simulink model "point_cloud_fusion_node_debag"  (R2021b)
settings: Solver=FixedStepAuto  StartTime=0.0  StopTime=10.0  RelTol=1e-3
model workspace (MAT data in the model file):
  Logfile_Data_Object = ros2bag
  Logfile_Data_Object.FilePath = 'C:\azumiken\lidars_point_raw\lidars_point_raw_0.db3'
  Logfile_Data_Object.StartTime = 1633675920681641206
  Logfile_Data_Object.EndTime = 1633676017682751873
  Logfile_Data_Object.AvailableTopics = table
  Logfile_Data_Object.AvailableTopics.data{1} = [969; 970]
  Logfile_Data_Object.AvailableTopics.data{2} = categorical
  Logfile_Data_Object.AvailableTopics.data{2}.categoryNames = {'sensor_msgs/PointCloud2'}
  Logfile_Data_Object.AvailableTopics.data{2}.codes = [1; 1]
  Logfile_Data_Object.AvailableTopics.data{3}{1} = '% contain additional information such as normals, intensity, etc. The
    | % point data is stored as a binary blob, its layout described by the
    | % contents of the "fields" array.
    | %
    | % The point cloud data may be organized 2d (image-like) or 1d (unordered).
    | % Point clouds organized as 2d images may be produced by camera depth sensors
    | % such as stereo or Time-of-flight.
    | 
    | % Time of sensor data acquisition, and the coordinate frame ID (for 3d points).
    | std_msgs/Header header
    | 
    | % 2D structure of the point cloud. If the cloud is unordered, height is
    | % 1 and width is the length of the point cloud.
    | uint32 height
    | uint32 width
    | 
    | % Describes the channels and their layout in the binary data blob.
    | PointField[] fields
    | 
    | logical    is_bigendian % Is this data bigendian?
    | uint32  point_step      % Length of a point in bytes
    | uint32  row_step        % Length of a row in bytes
    | uint8[] data            % Actual point data, size is (row_step*height)
    | 
    | logical is_dense        % True if there are no invalid points'
  Logfile_Data_Object.AvailableTopics.data{3}{2} = '% contain additional information such as normals, intensity, etc. The
    | % point data is stored as a binary blob, its layout described by the
    | % contents of the "fields" array.
    | %
    | % The point cloud data may be organized 2d (image-like) or 1d (unordered).
    | % Point clouds organized as 2d images may be produced by camera depth sensors
    | % such as stereo or Time-of-flight.
    | 
    | % Time of sensor data acquisition, and the coordinate frame ID (for 3d points).
    | std_msgs/Header header
    | 
    | % 2D structure of the point cloud. If the cloud is unordered, height is
    | % 1 and width is the length of the point cloud.
    | uint32 height
    | uint32 width
    | 
    | % Describes the channels and their layout in the binary data blob.
    | PointField[] fields
    | 
    | logical    is_bigendian % Is this data bigendian?
    | uint32  point_step      % Length of a point in bytes
    | uint32  row_step        % Length of a row in bytes
    | uint8[] data            % Actual point data, size is (row_step*height)
    | 
    | logical is_dense        % True if there are no invalid points'
  Logfile_Data_Object.AvailableTopics.ndims = 2
  Logfile_Data_Object.AvailableTopics.nrows = 2
  Logfile_Data_Object.AvailableTopics.rownames = {'/lidar_front/points_raw'; '/lidar_rear/points_raw'}
  Logfile_Data_Object.AvailableTopics.nvars = 3
  Logfile_Data_Object.AvailableTopics.varnames = {'NumMessages', 'MessageType', 'MessageDefinition'}
  Logfile_Data_Object.AvailableTopics.props.useVariableNamesOriginal = 0
  Logfile_Data_Object.AvailableTopics.props.useDimensionNamesOriginal = 0
  Logfile_Data_Object.AvailableTopics.props.CustomProps = struct()
  Logfile_Data_Object.AvailableTopics.props.VariableCustomProps = struct()
  Logfile_Data_Object.AvailableTopics.props.versionSavedFrom = 4
  Logfile_Data_Object.AvailableTopics.props.minCompatibleVersion = 1
  Logfile_Data_Object.AvailableTopics.props.incompatibilityMsg = ''
  Logfile_Data_Object.AvailableTopics.props.VersionSavedFrom = 4
  Logfile_Data_Object.AvailableTopics.props.Description = ''
  Logfile_Data_Object.AvailableTopics.props.VariableNamesOriginal = {}
  Logfile_Data_Object.AvailableTopics.props.DimensionNames = {'Row', 'Variables'}
  Logfile_Data_Object.AvailableTopics.props.DimensionNamesOriginal = {}
  Logfile_Data_Object.AvailableTopics.props.UserData = []
  Logfile_Data_Object.AvailableTopics.props.VariableDescriptions = {}
  Logfile_Data_Object.AvailableTopics.props.VariableUnits = {}
  Logfile_Data_Object.AvailableTopics.props.VariableContinuity = {}
  Logfile_Data_Object.MessageList = table
  Logfile_Data_Object.MessageList.data{1} = [1633675920681641206 1633675920704850047 1633675920710280571 1633675920841302537 1633675920849007917 1633675920944718285 1633675920950454411 1633675921046456357 1633675921051238695 1633675921143527086 1633675921154682295 1633675921262758351 ... (1939 elements, 1939x1)]
  Logfile_Data_Object.MessageList.data{2} = categorical
  Logfile_Data_Object.MessageList.data{2}.categoryNames = {'/lidar_rear/points_raw'; '/lidar_front/points_raw'}
  Logfile_Data_Object.MessageList.data{2}.codes = [1 2 1 2 1 2 1 2 1 2 1 2 ... (1939 elements, 1939x1)]
  Logfile_Data_Object.MessageList.data{3} = categorical
  Logfile_Data_Object.MessageList.data{3}.categoryNames = {'sensor_msgs/PointCloud2'}
  Logfile_Data_Object.MessageList.data{3}.codes = [1 1 1 1 1 1 1 1 1 1 1 1 ... (1939 elements, 1939x1)]
  Logfile_Data_Object.MessageList.ndims = 2
  Logfile_Data_Object.MessageList.nrows = 1939
  Logfile_Data_Object.MessageList.nvars = 3
  Logfile_Data_Object.MessageList.varnames = {'Time', 'Topic', 'MessageType'}
  Logfile_Data_Object.MessageList.props.useVariableNamesOriginal = 0
  Logfile_Data_Object.MessageList.props.useDimensionNamesOriginal = 0
  Logfile_Data_Object.MessageList.props.CustomProps = struct()
  Logfile_Data_Object.MessageList.props.VariableCustomProps = struct()
  Logfile_Data_Object.MessageList.props.versionSavedFrom = 4
  Logfile_Data_Object.MessageList.props.minCompatibleVersion = 1
  Logfile_Data_Object.MessageList.props.incompatibilityMsg = ''
  Logfile_Data_Object.MessageList.props.VersionSavedFrom = 4
  Logfile_Data_Object.MessageList.props.Description = ''
  Logfile_Data_Object.MessageList.props.VariableNamesOriginal = {}
  Logfile_Data_Object.MessageList.props.DimensionNames = {'Row', 'Variables'}
  Logfile_Data_Object.MessageList.props.DimensionNamesOriginal = {}
  Logfile_Data_Object.MessageList.props.UserData = []
  Logfile_Data_Object.MessageList.props.VariableDescriptions = {}
  Logfile_Data_Object.MessageList.props.VariableUnits = {}
  Logfile_Data_Object.MessageList.props.VariableContinuity = {}
  Logfile_Data_Object.TopicTypeMap = containers.Map
  Logfile_Data_Object.TopicTypeMap.serialization.keys = {'/lidar_front/points_raw', '/lidar_rear/points_raw'}
  Logfile_Data_Object.TopicTypeMap.serialization.values = {'sensor_msgs/PointCloud2', 'sensor_msgs/PointCloud2'}
  Logfile_Data_Object.TopicTypeMap.serialization.uniformity = 1
  Logfile_Data_Object.TopicTypeMap.serialization.keyType = 'char'
  Logfile_Data_Object.TopicTypeMap.serialization.valueType = 'char'
  Logfile_Data_Object.TopicDefinitionMap = containers.Map
  Logfile_Data_Object.TopicDefinitionMap.serialization.keys = {'/lidar_front/points_raw', '/lidar_rear/points_raw'}
  Logfile_Data_Object.TopicDefinitionMap.serialization.values{1} = '% contain additional information such as normals, intensity, etc. The
    | % point data is stored as a binary blob, its layout described by the
    | % contents of the "fields" array.
    | %
    | % The point cloud data may be organized 2d (image-like) or 1d (unordered).
    | % Point clouds organized as 2d images may be produced by camera depth sensors
    | % such as stereo or Time-of-flight.
    | 
    | % Time of sensor data acquisition, and the coordinate frame ID (for 3d points).
    | std_msgs/Header header
    | 
    | % 2D structure of the point cloud. If the cloud is unordered, height is
    | % 1 and width is the length of the point cloud.
    | uint32 height
    | uint32 width
    | 
    | % Describes the channels and their layout in the binary data blob.
    | PointField[] fields
    | 
    | logical    is_bigendian % Is this data bigendian?
    | uint32  point_step      % Length of a point in bytes
    | uint32  row_step        % Length of a row in bytes
    | uint8[] data            % Actual point data, size is (row_step*height)
    | 
    | logical is_dense        % True if there are no invalid points'
  Logfile_Data_Object.TopicDefinitionMap.serialization.values{2} = '% contain additional information such as normals, intensity, etc. The
    | % point data is stored as a binary blob, its layout described by the
    | % contents of the "fields" array.
    | %
    | % The point cloud data may be organized 2d (image-like) or 1d (unordered).
    | % Point clouds organized as 2d images may be produced by camera depth sensors
    | % such as stereo or Time-of-flight.
    | 
    | % Time of sensor data acquisition, and the coordinate frame ID (for 3d points).
    | std_msgs/Header header
    | 
    | % 2D structure of the point cloud. If the cloud is unordered, height is
    | % 1 and width is the length of the point cloud.
    | uint32 height
    | uint32 width
    | 
    | % Describes the channels and their layout in the binary data blob.
    | PointField[] fields
    | 
    | logical    is_bigendian % Is this data bigendian?
    | uint32  point_step      % Length of a point in bytes
    | uint32  row_step        % Length of a row in bytes
    | uint8[] data            % Actual point data, size is (row_step*height)
    | 
    | logical is_dense        % True if there are no invalid points'
  Logfile_Data_Object.TopicDefinitionMap.serialization.uniformity = 1
  Logfile_Data_Object.TopicDefinitionMap.serialization.keyType = 'char'
  Logfile_Data_Object.TopicDefinitionMap.serialization.valueType = 'char'
  Logfile_Path = 'C:\azumiken\lidars_point_raw\lidars_point_raw_0.db3'
  Logfile_Playback_Duration = nan
  Logfile_Playback_Offset = nan
  SL_ROS_VariableLengthArrays_MaxSizes.CommonInfo.ArrayTruncateAction = 'EmitWarning'
  SL_ROS_VariableLengthArrays_MaxSizes.MsgTypeMap = containers.Map
  SL_ROS_VariableLengthArrays_MaxSizes.MsgTypeMap.serialization.keys = {'sensor_msgs/PointCloud2'}
  SL_ROS_VariableLengthArrays_MaxSizes.MsgTypeMap.serialization.values{1}(1).PropertyName = 'data'
  SL_ROS_VariableLengthArrays_MaxSizes.MsgTypeMap.serialization.values{1}(1).DataType = 'uint8'
  SL_ROS_VariableLengthArrays_MaxSizes.MsgTypeMap.serialization.values{1}(1).MaxLength = 55000
  SL_ROS_VariableLengthArrays_MaxSizes.MsgTypeMap.serialization.values{1}(2).PropertyName = 'fields'
  SL_ROS_VariableLengthArrays_MaxSizes.MsgTypeMap.serialization.values{1}(2).DataType = 'sensor_msgs/PointField'
  SL_ROS_VariableLengthArrays_MaxSizes.MsgTypeMap.serialization.values{1}(2).MaxLength = 16
  SL_ROS_VariableLengthArrays_MaxSizes.MsgTypeMap.serialization.uniformity = 0
  SL_ROS_VariableLengthArrays_MaxSizes.MsgTypeMap.serialization.keyType = 'char'
  SL_ROS_VariableLengthArrays_MaxSizes.MsgTypeMap.serialization.valueType = 'any'
undefined symbols (not defined in the file or in its folder): data, header, height, row_step, width
libraries: ros2lib x9, simulink x4
settings Model: VariantFading=off  Creator=takum  LastModifiedBy=takum
settings SolverCC: AlgebraicLoopSolver=TrustRegion
settings OptimizationCC: EnhancedBackFolding=on  PassReuseOutputArgsAs=Individual arguments  ZeroExternalMemoryAtStartup=off  ZeroInternalMemoryAtStartup=off  MaxStackSize=64  OptimizeBlockOrder=speed  DifferentSizesBufferReuse=on  OptimizationCustomize=off  EfficientTunableParamExpr=on
settings DebuggingCC: ParameterTunabilityLossMsg=error  SFMachineParentedDataDiag=warning
settings SFSimCC: SimParseCustomCode=off  MATLABDynamicMemAlloc=off  SimTargetLang=C++
settings RTWCC: Description=Embedded Coder  SystemTargetFile=ert.tlc  HardwareBoard=Robot Operating System 2 (ROS 2)  TemplateMakefile=ert_default_tmf  Toolchain=Colcon Tools  TargetLang=C++
settings CodeAppCC: ForceParamTrailComments=on  IgnoreCustomStorageClasses=off  OperatorAnnotations=on  SimulinkDataObjDesc=on  SFDataObjDesc=on  InsertBlockDesc=on
settings ERTTargetCC: CodeInterfacePackaging=C++ class  RootIOFormat=Structure reference

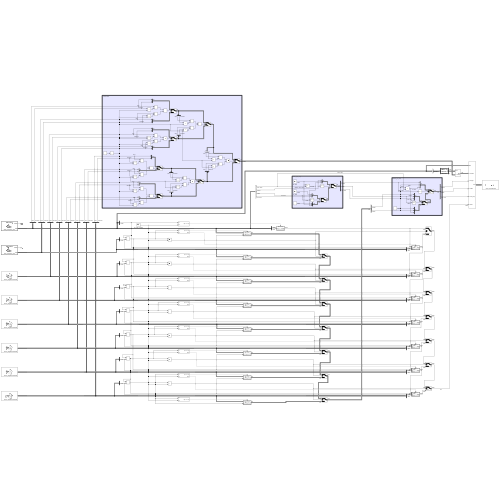
[thumbnail: Simulink's stored preview of the top-level diagram]
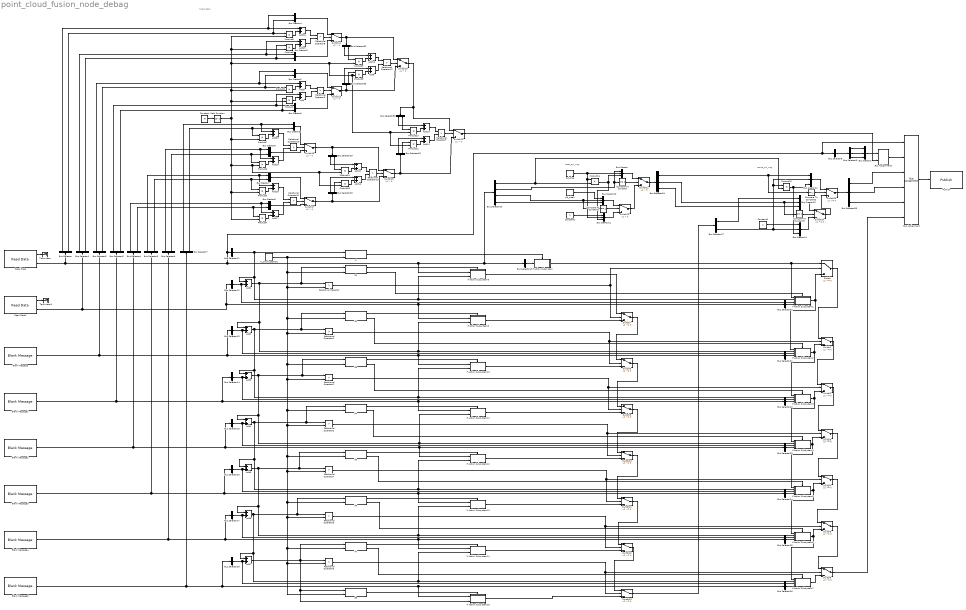
== system point_cloud_fusion_node_debag ==
  note: Subsystem
  note: reset_pcl_msg
  note: resize_pcl_msg
  Add{,1..20} (21 alike) : Sum
  Blank Message{,1..5} (6 alike) : ros2lib/Blank Message  messageClass=Message  entityType=sensor_msgs/PointCloud2  messageType=sensor_msgs/PointCloud2  SampleTime=inf
      settings: SourceProductBaseCode=RR
  Bus Assignment : BusAssignment  AssignedSignals=header,height,width,row_step,data
  Bus Assignment1 : BusAssignment  AssignedSignals=stamp
  Bus Creator{,1,10..14} (7 alike) : BusCreator  Inputs=3
  Bus Creator{2..9} (8 alike) : BusCreator  Inputs=2
  Bus Selector{,1..7} (8 alike) : BusSelector  OutputSignals=header.stamp.sec,header.stamp.nanosec
  Bus Selector10 : BusSelector  OutputSignals=point_step,height,width,row_step
  Bus Selector{11..18} (8 alike) : BusSelector  OutputSignals=width
  Bus Selector{19..26} (8 alike) : BusSelector  OutputSignals=data
  Bus Selector27 : BusSelector  OutputSignals=height,width
  Bus Selector{28..33} (6 alike) : BusSelector  OutputSignals=sec,nanosec
  Bus Selector34 : BusSelector  OutputSignals=height,width,row_step
  Bus Selector35 : BusSelector  OutputSignals=height,width,row_step
  Bus Selector8 : BusSelector  OutputSignals=header
  Bus Selector9 : BusSelector  OutputSignals=stamp,frame_id,frame_id_SL_Info
  Compare To Constant{,1..3} (4 alike) : simulink/Logic and Bit Operations/Compare To Constant  relop===  const=1  OutDataTypeStr=boolean
  Constant : Constant  Value=-9
  Constant1 : Constant
  Constant2 : Constant
  If : If  NumInputs=2  IfExpression=u1 <= u2  ShowElse=off
  If Action Subsystem : Subsystem  TreatAsAtomicUnit=on
  If Action Subsystem1 : Subsystem  TreatAsAtomicUnit=on
  If Action Subsystem10 : Subsystem  TreatAsAtomicUnit=on
  If Action Subsystem11 : Subsystem  TreatAsAtomicUnit=on
  If Action Subsystem12 : Subsystem  TreatAsAtomicUnit=on
  If Action Subsystem13 : Subsystem  TreatAsAtomicUnit=on
  If Action Subsystem14 : Subsystem  TreatAsAtomicUnit=on
  If Action Subsystem15 : Subsystem  TreatAsAtomicUnit=on
  If Action Subsystem2 : Subsystem  TreatAsAtomicUnit=on
  If Action Subsystem3 : Subsystem  TreatAsAtomicUnit=on
  If Action Subsystem4 : Subsystem  TreatAsAtomicUnit=on
  If Action Subsystem5 : Subsystem  TreatAsAtomicUnit=on
  If Action Subsystem6 : Subsystem  TreatAsAtomicUnit=on
  If Action Subsystem7 : Subsystem  TreatAsAtomicUnit=on
  If Action Subsystem8 : Subsystem  TreatAsAtomicUnit=on
  If Action Subsystem9 : Subsystem  TreatAsAtomicUnit=on
  If{1..7} (7 alike) : If  NumInputs=2  IfExpression=u1 > u2
  If8 : If  NumInputs=2  IfExpression=u1 <= u2  ShowElse=off
  Math Function : Math  Operator=10^u  SaturateOnIntegerOverflow=on
  Product{,1..15} (16 alike) : Product
  Publish : ros2lib/Publish  topicSource=Specify your own  topic=cloud_concatenated  messageType=sensor_msgs/PointCloud2  QOSHistory=Keep last  QOSDepth=1  QOSReliability=Reliable  QOSDurability=Volatile
      settings: SourceProductBaseCode=RR
  Read Data : ros2lib/Read Data  topic=/lidar_front/points_raw  sampleTime=-1  logfileType=rosbag2  modelName=point_cloud_fusion_node_debag  msgType=sensor_msgs/PointCloud2
      settings: SourceProductBaseCode=RR
  Read Data1 : ros2lib/Read Data  topic=/lidar_rear/points_raw  sampleTime=-1  logfileType=rosbag2  modelName=point_cloud_fusion_node_debag  msgType=sensor_msgs/PointCloud2
      settings: SourceProductBaseCode=RR
  Relational Operator{,1..13} (14 alike) : RelationalOperator  Operator=>  OutDataTypeStr=boolean  RndMeth=Simplest
  Switch{,1..13,23..24} (16 alike) : Switch  Criteria=u2 ~= 0
  Switch{14..22} (9 alike) : Switch  Criteria=u2 > Threshold
  Terminator : Terminator
  Terminator1 : Terminator
  m_cloud_capacity : Constant  Value=55000  OutDataTypeStr=uint32
  pcl_size : Constant  Value=55000
  pcl_size1 : Constant  Value=55000
  wires:
  Blank Message5/1 -> Bus Selector7/1, If Action Subsystem15/1(In1), Bus Selector26/1, Bus Selector18/1
  Blank Message4/1 -> Bus Selector6/1, If Action Subsystem14/1(In1), Bus Selector25/1, Bus Selector17/1
  Read Data1/2 -> Bus Selector1/1, If Action Subsystem9/1(In1), Bus Selector20/1, Bus Selector12/1
  Read Data1/1 -> Terminator1/1
  Blank Message/1 -> Bus Selector2/1, Bus Selector13/1, Bus Selector21/1, If Action Subsystem10/1(In1)
  Read Data/1 -> Terminator/1
  Blank Message2/1 -> Bus Selector4/1, Bus Selector23/1, If Action Subsystem12/1(In1), Bus Selector15/1
  If Action Subsystem6/1(msgs) -> If Action Subsystem7/1(In1), Switch5/3
  Bus Selector21/1 -> If Action Subsystem2/4(pc_in)  "<data>"
  Bus Selector5/1 -> Bus Creator7/1, Add18/1  "<sec>"
  Bus Creator4/1 -> Switch14/1
  Bus Selector3/1 -> Bus Creator9/1, Add/1  "<sec>"
  Bus Selector22/1 -> If Action Subsystem3/4(pc_in)  "<data>"
  Bus Selector3/2 -> Bus Creator9/2, Product/1  "<nanosec>"
  Bus Selector27/1 -> Bus Creator13/1  "<height>"
  Bus Selector35/3 -> Bus Assignment/5  "<row_step>"
  Switch10/1 -> Switch11/1
  Switch16/1 -> Switch19/1, Bus Selector28/1
  Bus Selector13/1 -> If Action Subsystem2/3(In3), Add2/2  "<width>"
  Add1/1 -> If Action Subsystem9/2(In2), If Action Subsystem2/2(<width>), Add2/1, Relational Operator/1, If1/1
  pcl_size1/1 -> Bus Creator10/1  "height"
  Switch13/1 -> Bus Selector27/1
  Switch14/1 -> Switch18/1, Bus Selector32/1
  If/1 -> If Action Subsystem/Action
  Bus Selector17/1 -> If Action Subsystem6/3(In3), Add6/2  "<width>"
  Switch5/1 -> Switch6/1
  If Action Subsystem10/1(Out1) -> Switch8/3
  Relational Operator10/1 -> Switch16/2
  If Action Subsystem14/1(Out1) -> Switch12/3
  Relational Operator1/1 -> Switch8/2, Switch1/2
  Read Data/2 -> Bus Selector/1, Bus Selector11/1, Bus Assignment/1, Bus Selector8/1, Bus Selector19/1, Bus Selector10/1, If Action Subsystem8/1(In1)
  If8/1 -> If Action Subsystem15/Action
  If Action Subsystem15/1(Out1) -> Switch13/3
  Bus Selector30/1 -> Add13/1  "<sec>"
  Bus Selector16/1 -> If Action Subsystem5/3(In3), Add5/2  "<width>"
  If6/1 -> If Action Subsystem13/Action
  Add7/1 -> If8/1, If Action Subsystem15/2(In2), If7/1, Relational Operator6/1
  Bus Selector26/1 -> If Action Subsystem7/4(pc_in)  "<data>"
  Switch8/1 -> Switch9/1
  Bus Selector/2 -> Product3/1, Bus Creator4/2  "<nanosec>"
  Blank Message3/1 -> Bus Selector5/1, Bus Selector24/1, If Action Subsystem13/1(In1), Bus Selector16/1
  m_cloud_capacity/1 -> Relational Operator3/2, Relational Operator4/2, If8/2, Relational Operator6/2, If7/2, Relational Operator5/2, If6/2, If5/2, If4/2, Relational Operator2/2, If3/2, Relational Operator1/2, If2/2, Relational Operator/2, If1/2, If/2
  Bus Selector10/3 -> Compare To Constant1/1, Bus Creator10/2  "<width>"
  Bus Selector32/2 -> Product9/1  "<nanosec>"
  Switch7/1 -> Switch8/1
  Add10/1 -> Relational Operator12/1
  Compare To Constant3/1 -> Switch24/2
  Bus Selector8/1 -> Bus Selector9/1  "<header>"
  Bus Selector5/2 -> Bus Creator7/2, Product5/1  "<nanosec>"
  Bus Selector31/1 -> Add14/1  "<sec>"
  Bus Selector14/1 -> If Action Subsystem3/3(In3), Add3/2  "<width>"
  Switch17/1 -> Switch19/3, Bus Selector29/1
  Bus Selector29/2 -> Product10/1  "<nanosec>"
  Add12/1 -> Relational Operator13/2
  Add6/1 -> If Action Subsystem14/2(In2), If Action Subsystem7/2(<width>), Add7/1, If6/1, Relational Operator5/1
  Add11/1 -> Relational Operator13/1
  Bus Creator1/1 -> Bus Assignment1/1
  Bus Selector20/1 -> If Action Subsystem1/4(pc_in)  "<data>"
  Bus Creator10/1 -> Switch22/1
  Bus Selector33/2 -> Product8/1  "<nanosec>"
  Add20/1 -> Relational Operator10/1
  Add19/1 -> Relational Operator10/2
  Switch1/1 -> Switch2/1
  Switch22/1 -> Switch21/3
  If Action Subsystem3/1(msgs) -> If Action Subsystem4/1(In1), Switch2/3
  Switch4/1 -> Switch5/1
  If7/1 -> If Action Subsystem14/Action
  Bus Selector9/2 -> Bus Creator1/2  "<frame_id>"
  Product13/1 -> Add13/2
  Bus Selector/1 -> Add16/1, Bus Creator4/1  "<sec>"
  If5/2 -> If Action Subsystem5/Action
  Bus Assignment1/1 -> Bus Assignment/2
  Relational Operator5/1 -> Switch12/2, Switch5/2
  If Action Subsystem13/1(Out1) -> Switch11/3
  Add9/1 -> Relational Operator12/2
  Bus Creator14/1 -> Switch24/3
  Add8/1 -> Relational Operator9/1
  Bus Selector31/2 -> Product12/1  "<nanosec>"
  If4/2 -> If Action Subsystem4/Action
  Product12/1 -> Add14/2
  Switch3/1 -> Switch4/1
  Product4/1 -> Add17/2
  Switch19/1 -> Bus Selector31/1, Switch20/3
  Bus Selector29/1 -> Add12/1  "<sec>"
  Switch/1 -> Switch1/1
  Product11/1 -> Add11/2
  pcl_size/1 -> Bus Creator/2, Bus Creator11/2, Product14/1  "width"
  Bus Creator13/1 -> Switch24/1
  Relational Operator9/1 -> Switch15/2
  Bus Selector30/2 -> Product13/1  "<nanosec>"
  Bus Selector7/2 -> Bus Creator5/2, Product7/1  "<nanosec>"
  If Action Subsystem/1(msgs) -> If Action Subsystem1/1(In1), Switch/1
  Product3/1 -> Add16/2
  Bus Selector28/1 -> Add11/1  "<sec>"
  Bus Selector9/1 -> Bus Creator1/1  "<stamp>"
  If6/2 -> If Action Subsystem6/Action
  Bus Selector35/1 -> Bus Assignment/3  "<height>"
  If Action Subsystem11/1(Out1) -> Switch9/3
  Switch9/1 -> Switch10/1
  Constant/1 -> Math Function/1
  Bus Selector32/1 -> Add10/1  "<sec>"
  If1/1 -> If Action Subsystem8/Action
  If2/2 -> If Action Subsystem2/Action
  If3/1 -> If Action Subsystem10/Action
  Add/1 -> Relational Operator9/2
  Bus Creator12/1 -> Switch23/1
  Bus Selector7/1 -> Add20/1, Bus Creator5/1  "<sec>"
  If7/2 -> If Action Subsystem7/Action
  Constant2/1 -> Bus Creator14/1  "height"
  Bus Creator6/1 -> Switch16/3
  Bus Creator11/1 -> Switch22/3
  Product6/1 -> Add19/2
  Bus Selector2/1 -> Bus Creator2/1, Add8/1  "<sec>"
  Bus Selector28/2 -> Product11/1  "<nanosec>"
  Product2/1 -> Add15/2
  Compare To Constant2/1 -> Switch23/2
  Relational Operator7/1 -> Switch20/2
  Bus Selector33/1 -> Add9/1  "<sec>"
  Product/1 -> Add/2
  Add15/1 -> Relational Operator8/2
  If Action Subsystem2/1(msgs) -> If Action Subsystem3/1(In1), Switch1/3
  Compare To Constant/1 -> Switch21/2
  Add4/1 -> If Action Subsystem12/2(In2), If Action Subsystem5/2(<width>), Add5/1, If4/1, Relational Operator3/1
  Add3/1 -> If3/1, Relational Operator2/1, Add4/1, If Action Subsystem4/2(<width>), If Action Subsystem11/2(In2)
  Bus Selector34/2 -> Compare To Constant3/1, Bus Creator13/2  "<width>"
  Bus Creator9/1 -> Switch15/3
  Add14/1 -> Relational Operator7/2
  Relational Operator2/1 -> Switch2/2, Switch9/2
  If2/1 -> If Action Subsystem9/Action
  Product15/1 -> Bus Creator12/3, Bus Creator14/3  "row_step"
  Switch21/1 -> Bus Selector34/1
  Add18/1 -> Relational Operator11/1
  Product1/1 -> Add8/2
  Product14/1 -> Bus Creator11/3, Bus Creator/3  "row_step"
  Switch12/1 -> Switch13/1
  Bus Assignment/1 -> Publish/1
  Switch20/1 -> Bus Assignment1/2  "header.stamp"
  Bus Selector11/1 -> If Action Subsystem1/2(<width>), If Action Subsystem8/2(In2), Add1/1, If/1  "<width>"
  Product5/1 -> Add18/2
  Bus Selector34/1 -> Compare To Constant2/1, Bus Creator12/1  "<height>"
  Add17/1 -> Relational Operator11/2
  Bus Creator/1 -> Switch21/1
  Product9/1 -> Add10/2
  If Action Subsystem7/1(msgs) -> Switch6/3
  Bus Creator2/1 -> Switch15/1
  Bus Selector23/1 -> If Action Subsystem4/4(pc_in)  "<data>"
  Constant1/1 -> Bus Creator11/1  "height"
  Relational Operator8/1 -> Switch14/2
  If Action Subsystem1/1(msgs) -> Switch/3, If Action Subsystem2/1(In1)
  Add13/1 -> Relational Operator7/1
  Switch2/1 -> Switch3/1
  Product8/1 -> Add9/2
  Switch15/1 -> Bus Selector33/1, Switch18/3
  Blank Message1/1 -> Bus Selector3/1, If Action Subsystem11/1(In1), Bus Selector22/1, Bus Selector14/1
  Bus Selector25/1 -> If Action Subsystem6/4(pc_in)  "<data>"
  Bus Selector6/2 -> Bus Creator6/2, Product6/1  "<nanosec>"
  Add16/1 -> Relational Operator8/1
  Product10/1 -> Add12/2
  Bus Selector10/2 -> Bus Creator/1, Compare To Constant/1  "<height>"
  Math Function/1 -> Product4/2, Product5/2, Product10/2, Product11/2, Product6/2, Product7/2, Product2/2, Product3/2, Product13/2, Product12/2, Product8/2, Product9/2, Product1/2, Product/2
  Bus Creator3/1 -> Switch14/3
  If Action Subsystem12/1(Out1) -> Switch10/3
  Bus Selector15/1 -> If Action Subsystem4/3(In3), Add4/2  "<width>"
  Relational Operator3/1 -> Switch10/2, Switch3/2
  Bus Selector12/1 -> If Action Subsystem1/3(In3), Add1/2  "<width>"
  Bus Selector34/3 -> Bus Creator13/3  "<row_step>"
  Bus Selector9/3 -> Bus Creator1/3  "<frame_id_SL_Info>"
  Relational Operator4/1 -> Switch11/2, Switch4/2
  Bus Selector4/2 -> Bus Creator8/2, Product4/1  "<nanosec>"
  Bus Selector35/2 -> Bus Assignment/4  "<width>"
  If4/1 -> If Action Subsystem11/Action
  Relational Operator13/1 -> Switch19/2
  Product7/1 -> Add20/2
  If Action Subsystem5/1(msgs) -> If Action Subsystem6/1(In1), Switch4/3
  Compare To Constant1/1 -> Switch22/2
  Relational Operator6/1 -> Switch13/2, Switch6/2
  Bus Creator7/1 -> Switch17/1
  Relational Operator11/1 -> Switch17/2
  If Action Subsystem9/1(Out1) -> Switch7/3
  If Action Subsystem8/1(Out1) -> Switch7/1
  Bus Selector18/1 -> If Action Subsystem7/3(In3), Add7/2  "<width>"
  Bus Selector1/1 -> Add15/1, Bus Creator3/1  "<sec>"
  Switch23/1 -> Bus Selector35/1
  Bus Selector2/2 -> Bus Creator2/2, Product1/1  "<nanosec>"
  Switch6/1 -> Bus Assignment/6  "data"
  Bus Creator5/1 -> Switch16/1
  Relational Operator12/1 -> Switch18/2
  If3/2 -> If Action Subsystem3/Action
  Bus Selector4/1 -> Bus Creator8/1, Add17/1  "<sec>"
  Bus Selector24/1 -> If Action Subsystem5/4(pc_in)  "<data>"
  If1/2 -> If Action Subsystem1/Action
  Bus Selector6/1 -> Add19/1, Bus Creator6/1  "<sec>"
  Bus Selector27/2 -> Bus Creator12/2, Product15/1, Bus Creator14/2  "<width>"
  If5/1 -> If Action Subsystem12/Action
  Bus Selector1/2 -> Product2/1, Bus Creator3/2  "<nanosec>"
  Bus Selector10/4 -> Bus Creator10/3  "<row_step>"
  If Action Subsystem4/1(msgs) -> If Action Subsystem5/1(In1), Switch3/3
  Bus Selector10/1 -> Product15/2, Product14/2  "<point_step>"
  Switch18/1 -> Bus Selector30/1, Switch20/1
  Switch24/1 -> Switch23/3
  Bus Selector19/1 -> If Action Subsystem/1(pc_in)  "<data>"
  Relational Operator/1 -> Switch/2, Switch7/2
  Bus Creator8/1 -> Switch17/3
  Add5/1 -> If5/1, Relational Operator4/1, If Action Subsystem13/2(In2), If Action Subsystem6/2(<width>), Add6/1
  Switch11/1 -> Switch12/1
  Add2/1 -> If2/1, Relational Operator1/1, If Action Subsystem10/2(In2), If Action Subsystem3/2(<width>), Add3/1

== system point_cloud_fusion_node_debag/If Action Subsystem ==
  pc_in : Inport
  Action Port : ActionPort  ActionPortLabel=if(u1 <= u2)
  msgs : Outport
  wires:
  pc_in/1 -> msgs/1

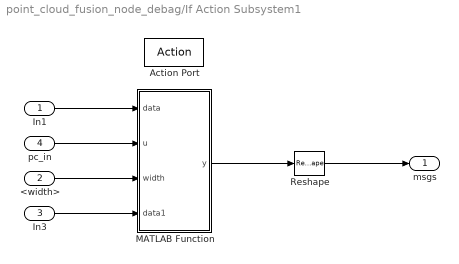
== system point_cloud_fusion_node_debag/If Action Subsystem1 ==
  In1 : Inport
  <width> : Inport  Port=2
  In3 : Inport  Port=3
  pc_in : Inport  Port=4
  Action Port : ActionPort  ActionPortLabel=else
  MATLAB Function : MATLAB Function  TreatAsAtomicUnit=on
  Reshape : Reshape
  msgs : Outport
  wires:
  pc_in/1 -> MATLAB Function/2(u)
  MATLAB Function/1(y) -> Reshape/1
  In1/1 -> MATLAB Function/1(data)
  <width>/1 -> MATLAB Function/3(width)
  In3/1 -> MATLAB Function/4(data1)
  Reshape/1 -> msgs/1

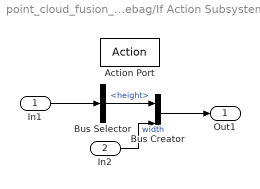
== system point_cloud_fusion_node_debag/If Action Subsystem10 ==
  In1 : Inport
  In2 : Inport  Port=2
  Action Port : ActionPort  ActionPortLabel=if(u1 > u2)
  Bus Creator : BusCreator  Inputs=2
  Bus Selector : BusSelector  OutputSignals=height
  Out1 : Outport
  wires:
  In1/1 -> Bus Selector/1
  Bus Selector/1 -> Bus Creator/1  "<height>"
  Bus Creator/1 -> Out1/1
  In2/1 -> Bus Creator/2  "width"

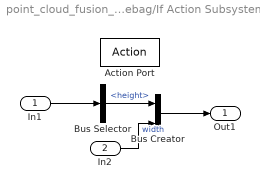
== system point_cloud_fusion_node_debag/If Action Subsystem11 ==
  In1 : Inport
  In2 : Inport  Port=2
  Action Port : ActionPort  ActionPortLabel=if(u1 > u2)
  Bus Creator : BusCreator  Inputs=2
  Bus Selector : BusSelector  OutputSignals=height
  Out1 : Outport
  wires:
  In1/1 -> Bus Selector/1
  Bus Selector/1 -> Bus Creator/1  "<height>"
  Bus Creator/1 -> Out1/1
  In2/1 -> Bus Creator/2  "width"

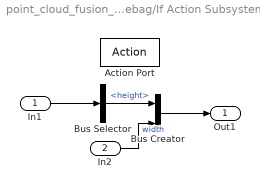
== system point_cloud_fusion_node_debag/If Action Subsystem12 ==
  In1 : Inport
  In2 : Inport  Port=2
  Action Port : ActionPort  ActionPortLabel=if(u1 > u2)
  Bus Creator : BusCreator  Inputs=2
  Bus Selector : BusSelector  OutputSignals=height
  Out1 : Outport
  wires:
  In1/1 -> Bus Selector/1
  Bus Selector/1 -> Bus Creator/1  "<height>"
  Bus Creator/1 -> Out1/1
  In2/1 -> Bus Creator/2  "width"

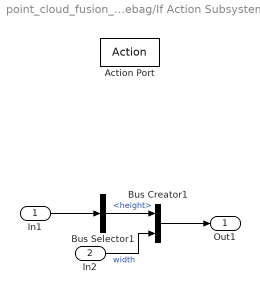
== system point_cloud_fusion_node_debag/If Action Subsystem13 ==
  In1 : Inport
  In2 : Inport  Port=2
  Action Port : ActionPort  ActionPortLabel=if(u1 > u2)
  Bus Creator1 : BusCreator  Inputs=2
  Bus Selector1 : BusSelector  OutputSignals=height
  Out1 : Outport
  wires:
  Bus Creator1/1 -> Out1/1
  In2/1 -> Bus Creator1/2  "width"
  Bus Selector1/1 -> Bus Creator1/1  "<height>"
  In1/1 -> Bus Selector1/1

== system point_cloud_fusion_node_debag/If Action Subsystem14 ==
  In1 : Inport
  In2 : Inport  Port=2
  Action Port : ActionPort  ActionPortLabel=if(u1 > u2)
  Bus Creator : BusCreator  Inputs=2
  Bus Selector : BusSelector  OutputSignals=height
  Out1 : Outport
  wires:
  In1/1 -> Bus Selector/1
  Bus Selector/1 -> Bus Creator/1  "<height>"
  Bus Creator/1 -> Out1/1
  In2/1 -> Bus Creator/2  "width"

== system point_cloud_fusion_node_debag/If Action Subsystem15 ==
  In1 : Inport
  In2 : Inport  Port=2
  Action Port : ActionPort  ActionPortLabel=if(u1 <= u2)
  Bus Creator : BusCreator  Inputs=2
  Bus Selector : BusSelector  OutputSignals=height
  Out1 : Outport
  wires:
  In1/1 -> Bus Selector/1
  Bus Selector/1 -> Bus Creator/1  "<height>"
  Bus Creator/1 -> Out1/1
  In2/1 -> Bus Creator/2  "width"

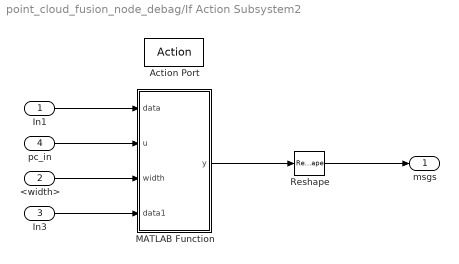
== system point_cloud_fusion_node_debag/If Action Subsystem2 ==
  In1 : Inport
  <width> : Inport  Port=2
  In3 : Inport  Port=3
  pc_in : Inport  Port=4
  Action Port : ActionPort  ActionPortLabel=else
  MATLAB Function : MATLAB Function  TreatAsAtomicUnit=on
  Reshape : Reshape
  msgs : Outport
  wires:
  pc_in/1 -> MATLAB Function/2(u)
  MATLAB Function/1(y) -> Reshape/1
  In1/1 -> MATLAB Function/1(data)
  <width>/1 -> MATLAB Function/3(width)
  In3/1 -> MATLAB Function/4(data1)
  Reshape/1 -> msgs/1

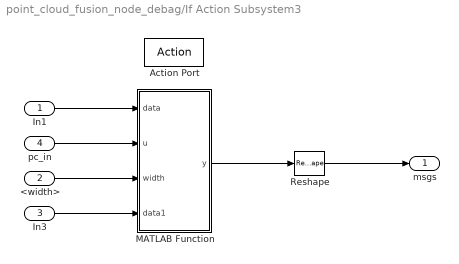
== system point_cloud_fusion_node_debag/If Action Subsystem3 ==
  In1 : Inport
  <width> : Inport  Port=2
  In3 : Inport  Port=3
  pc_in : Inport  Port=4
  Action Port : ActionPort  ActionPortLabel=else
  MATLAB Function : MATLAB Function  TreatAsAtomicUnit=on
  Reshape : Reshape
  msgs : Outport
  wires:
  pc_in/1 -> MATLAB Function/2(u)
  MATLAB Function/1(y) -> Reshape/1
  In1/1 -> MATLAB Function/1(data)
  <width>/1 -> MATLAB Function/3(width)
  In3/1 -> MATLAB Function/4(data1)
  Reshape/1 -> msgs/1

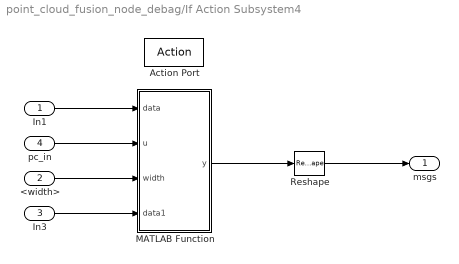
== system point_cloud_fusion_node_debag/If Action Subsystem4 ==
  In1 : Inport
  <width> : Inport  Port=2
  In3 : Inport  Port=3
  pc_in : Inport  Port=4
  Action Port : ActionPort  ActionPortLabel=else
  MATLAB Function : MATLAB Function  TreatAsAtomicUnit=on
  Reshape : Reshape
  msgs : Outport
  wires:
  pc_in/1 -> MATLAB Function/2(u)
  MATLAB Function/1(y) -> Reshape/1
  In1/1 -> MATLAB Function/1(data)
  <width>/1 -> MATLAB Function/3(width)
  In3/1 -> MATLAB Function/4(data1)
  Reshape/1 -> msgs/1

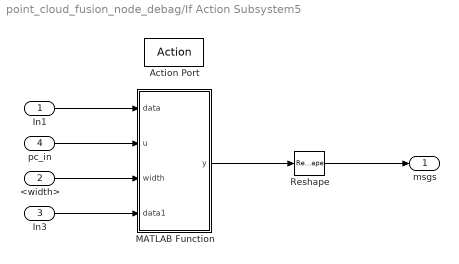
== system point_cloud_fusion_node_debag/If Action Subsystem5 ==
  In1 : Inport
  <width> : Inport  Port=2
  In3 : Inport  Port=3
  pc_in : Inport  Port=4
  Action Port : ActionPort  ActionPortLabel=else
  MATLAB Function : MATLAB Function  TreatAsAtomicUnit=on
  Reshape : Reshape
  msgs : Outport
  wires:
  pc_in/1 -> MATLAB Function/2(u)
  MATLAB Function/1(y) -> Reshape/1
  In1/1 -> MATLAB Function/1(data)
  <width>/1 -> MATLAB Function/3(width)
  In3/1 -> MATLAB Function/4(data1)
  Reshape/1 -> msgs/1

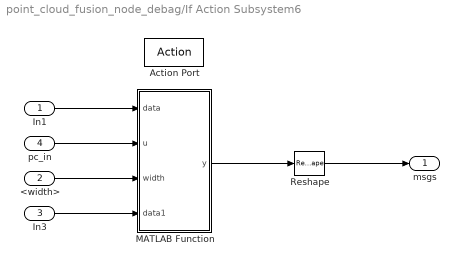
== system point_cloud_fusion_node_debag/If Action Subsystem6 ==
  In1 : Inport
  <width> : Inport  Port=2
  In3 : Inport  Port=3
  pc_in : Inport  Port=4
  Action Port : ActionPort  ActionPortLabel=else
  MATLAB Function : MATLAB Function  TreatAsAtomicUnit=on
  Reshape : Reshape
  msgs : Outport
  wires:
  pc_in/1 -> MATLAB Function/2(u)
  MATLAB Function/1(y) -> Reshape/1
  In1/1 -> MATLAB Function/1(data)
  <width>/1 -> MATLAB Function/3(width)
  In3/1 -> MATLAB Function/4(data1)
  Reshape/1 -> msgs/1

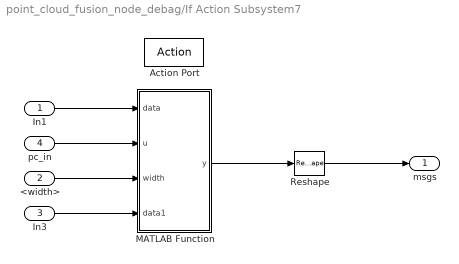
== system point_cloud_fusion_node_debag/If Action Subsystem7 ==
  In1 : Inport
  <width> : Inport  Port=2
  In3 : Inport  Port=3
  pc_in : Inport  Port=4
  Action Port : ActionPort  ActionPortLabel=else
  MATLAB Function : MATLAB Function  TreatAsAtomicUnit=on
  Reshape : Reshape
  msgs : Outport
  wires:
  pc_in/1 -> MATLAB Function/2(u)
  MATLAB Function/1(y) -> Reshape/1
  In1/1 -> MATLAB Function/1(data)
  <width>/1 -> MATLAB Function/3(width)
  In3/1 -> MATLAB Function/4(data1)
  Reshape/1 -> msgs/1

== system point_cloud_fusion_node_debag/If Action Subsystem8 ==
  In1 : Inport
  In2 : Inport  Port=2
  Action Port : ActionPort  ActionPortLabel=if(u1 > u2)
  Bus Creator : BusCreator  Inputs=2
  Bus Selector : BusSelector  OutputSignals=height
  Out1 : Outport
  wires:
  In1/1 -> Bus Selector/1
  Bus Selector/1 -> Bus Creator/1  "<height>"
  Bus Creator/1 -> Out1/1
  In2/1 -> Bus Creator/2  "width"

== system point_cloud_fusion_node_debag/If Action Subsystem9 ==
  In1 : Inport
  In2 : Inport  Port=2
  Action Port : ActionPort  ActionPortLabel=if(u1 > u2)
  Bus Creator : BusCreator  Inputs=2
  Bus Selector : BusSelector  OutputSignals=height
  Out1 : Outport
  wires:
  In1/1 -> Bus Selector/1
  Bus Selector/1 -> Bus Creator/1  "<height>"
  Bus Creator/1 -> Out1/1
  In2/1 -> Bus Creator/2  "width"

== matlab function point_cloud_fusion_node_debag/If Action Subsystem2/MATLAB Function ==
  data: data input; u input; y output; width input; data1 input
function y = fcn(data, u, width, data1)
s=width+1;
f=width+data1;
data(s:f)=u(1:data1);
y=data;

== matlab function point_cloud_fusion_node_debag/If Action Subsystem1/MATLAB Function ==
  data: data input; u input; y output; width input; data1 input
function y = fcn(data, u, width, data1)
s=width+1;
f=width+data1;
data(s:f)=u(1:data1);
y=data;

== matlab function point_cloud_fusion_node_debag/If Action Subsystem3/MATLAB Function ==
  data: data input; u input; y output; width input; data1 input
function y = fcn(data, u, width, data1)
s=width+1;
f=width+data1;
data(s:f)=u(1:data1);
y=data;

== matlab function point_cloud_fusion_node_debag/If Action Subsystem4/MATLAB Function ==
  data: data input; u input; y output; width input; data1 input
function y = fcn(data, u, width, data1)
s=width+1;
f=width+data1;
data(s:f)=u(1:data1);
y=data;

== matlab function point_cloud_fusion_node_debag/If Action Subsystem5/MATLAB Function ==
  data: data input; u input; y output; width input; data1 input
function y = fcn(data, u, width, data1)
s=width+1;
f=width+data1;
data(s:f)=u(1:data1);
y=data;

== matlab function point_cloud_fusion_node_debag/If Action Subsystem6/MATLAB Function ==
  data: data input; u input; y output; width input; data1 input
function y = fcn(data, u, width, data1)
s=width+1;
f=width+data1;
data(s:f)=u(1:data1);
y=data;

== matlab function point_cloud_fusion_node_debag/If Action Subsystem7/MATLAB Function ==
  data: data input; u input; y output; width input; data1 input
function y = fcn(data, u, width, data1)
s=width+1;
f=width+data1;
data(s:f)=u(1:data1);
y=data;
